simulink model "schiefer_wurf"  (R2025b)
settings: Solver=ode45  StartTime=0.0  StopTime=t_end  RelTol=1e-3
undefined symbols (not defined in the file): g, km, vx0, vy0, x0, y0
libraries: simulink x2
settings Model: Creator=arash  LastModifiedBy=arash

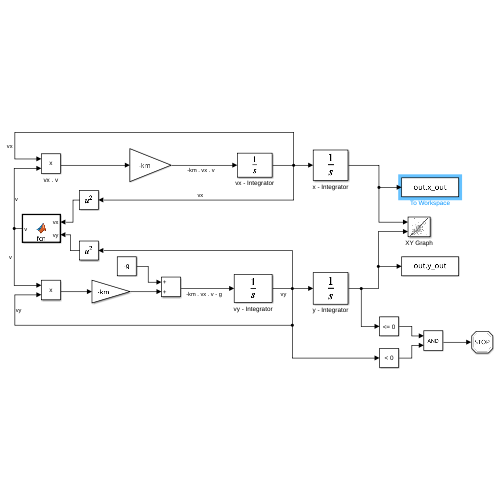
[thumbnail: Simulink's stored preview of the top-level diagram]
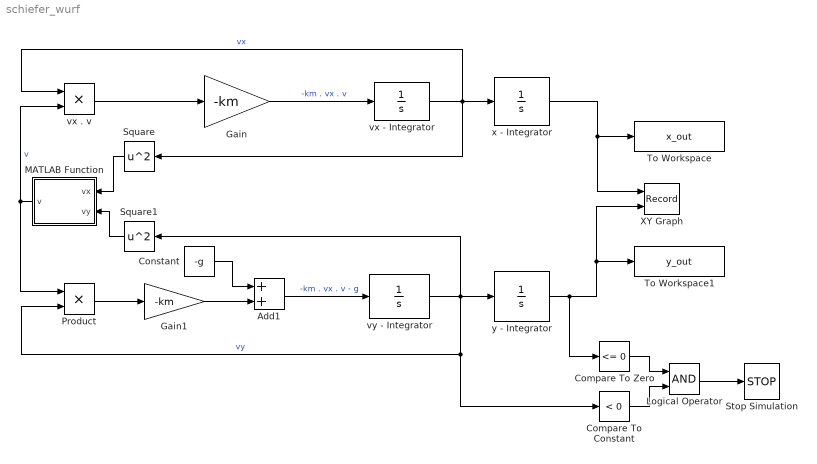
== system schiefer_wurf ==
  Add1 : Sum
  Compare To Constant : simulink/Logic and Bit Operations/Compare To Constant  relop=<  const=0  OutDataTypeStr=boolean
  Compare To Zero : simulink/Logic and Bit Operations/Compare To Zero  relop=<=  OutDataTypeStr=boolean
  Constant : Constant  Value=-g
  Gain : Gain  Gain=-km
  Gain1 : Gain  Gain=-km
  Logical Operator : Logic  AllPortsSameDT=off  OutDataTypeStr=boolean
  MATLAB Function : MATLAB Function  TreatAsAtomicUnit=on
  Product : Product
  Square : Math  Operator=square
  Square1 : Math  Operator=square
  Stop Simulation : Stop
  To Workspace : ToWorkspace  VariableName=x_out  SampleTime=-1
  To Workspace1 : ToWorkspace  VariableName=y_out  SampleTime=-1
  XY Graph : Record  NumPorts=2.0  FileSettingsInternal="{\"entries\":[{\"content\":{\"excelSettings\":{\"content\":{},\"type\":\"Streamout.ExcelSettings\"},\"parquetSettings\":{\"content\":{},\"type\":\"Streamout.ParquetSettings\"}},\"type\":\"Streamout.FileSettingStorage\",\"uuid\":\"\"}],\"packageUris\":[\"http:\\/\\/schema.mathworks.com\\/mf0\\/streamout_blocks\\/R2020a\"],\"version\":\"1.0\"}"  FrameSettings=[0, 0]  Layout=[1 1]  SignalsInternal="{\"entries\":[{\"content\":{\"signals\":[{\"content\":{\"blockPath\":[],\"dimensions\":[1],\"domain\":\"\",\"lineColor\":\"#a2142f\",\"plots\":[ 1 ],\"port\":1,\"sid\":[\"\"],\"signalID\":1,\"signalName\":\"x - Integrator\"},\"type\":\"RecordBlkView.Signal\",\"uuid\":\"\"},{\"content\":{\"blockPath\":[],\"dimensions\":[1],\"domain\":\"\",\"lineColor\":\"#139fff\",\"plots\":[ 1 ],\"port\":2,\"sid\":[\"\"],\"signalID\":2,\"signalName\":\"y - Integrator\"},\"type\":\"RecordBlkView.Signal\",\"uuid\":\"\"}]},\"type\":\"RecordBlkView.InputSignals\",\"uuid\":\"\"}],\"packageUris\":[\"http:\\/\\/schema.mathworks.com\\/mf0\\/streamout_blocks\\/R2020a\"],\"version\":\"1.0\"}"  VisualizationBindings="{\"xyplotplugin\":{\"info\":[{\"series\":[{\"bindingParametersList\":[{\"parameter\":\"X-Axis\",\"signalID\":1,\"signalName\":\"x - Integrator\"},{\"parameter\":\"Y-Axis\",\"signalID\":2,\"signalName\":\"y - Integrator\"}],\"seriesID\":0}],\"subplotID\":1}]}}"  CompatibilityTag=XY
  vx - Integrator : Integrator  InitialCondition=vx0
  vx . v : Product
  vy - Integrator : Integrator  InitialCondition=vy0
  x - Integrator : Integrator  InitialCondition=x0
  y - Integrator : Integrator  InitialCondition=y0
  wires:
  Gain/1 -> vx - Integrator/1  "-km . vx . v"
  vy - Integrator/1 -> Compare To Constant/1, Product/2, Square1/1, y - Integrator/1  "vy"
  Square/1 -> MATLAB Function/1(vx)
  Square1/1 -> MATLAB Function/2(vy)
  MATLAB Function/1(v) -> Product/1, vx . v/2  "v"
  vx - Integrator/1 -> x - Integrator/1, Square/1, vx . v/1  "vx"
  vx . v/1 -> Gain/1
  Product/1 -> Gain1/1
  Gain1/1 -> Add1/2
  Constant/1 -> Add1/1
  Add1/1 -> vy - Integrator/1  "-km . vx . v - g"
  x - Integrator/1 -> XY Graph/1, To Workspace/1
  y - Integrator/1 -> Compare To Zero/1, To Workspace1/1, XY Graph/2
  Compare To Zero/1 -> Logical Operator/1
  Compare To Constant/1 -> Logical Operator/2
  Logical Operator/1 -> Stop Simulation/1

== matlab function schiefer_wurf/MATLAB Function ==
  data: vx input; v output; vy input
function v = fcn(vx,vy)

v = sqrt(vx^2 + vy^2);
